simulink model "svm_Filter"  (R2023b)
settings: Solver=FixedStepAuto  StartTime=0.0  StopTime=0.08  FixedStep=0.5e-7  RelTol=1e-3
InitFcn:
  | TP=0.0002
  | Vdc=580
undefined symbols (not defined in the file): Ma
libraries: spsMosfetLib x6, spsSeriesRLCBranchLib x3, spsVoltageMeasurementLib x3, spsDCVoltageSourceLib x1, spsGroundLib x1, spsThreePhaseVIMeasurementLib x1, sps_lib x1, mcbcontrolslib x1, simulink_extras x1
settings Model: Creator=user  LastModifiedBy=user
settings DataIOCC: ReturnWorkspaceOutputs=off

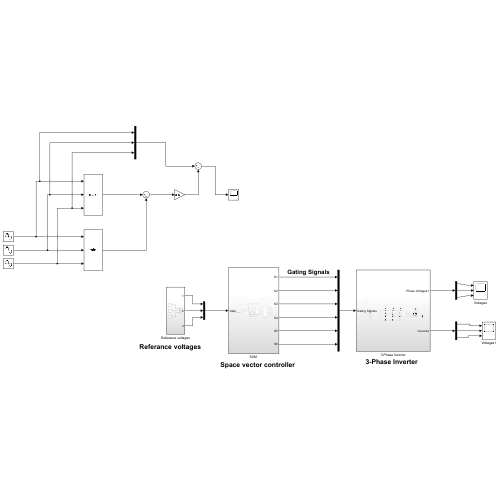
[thumbnail: Simulink's stored preview of the top-level diagram]
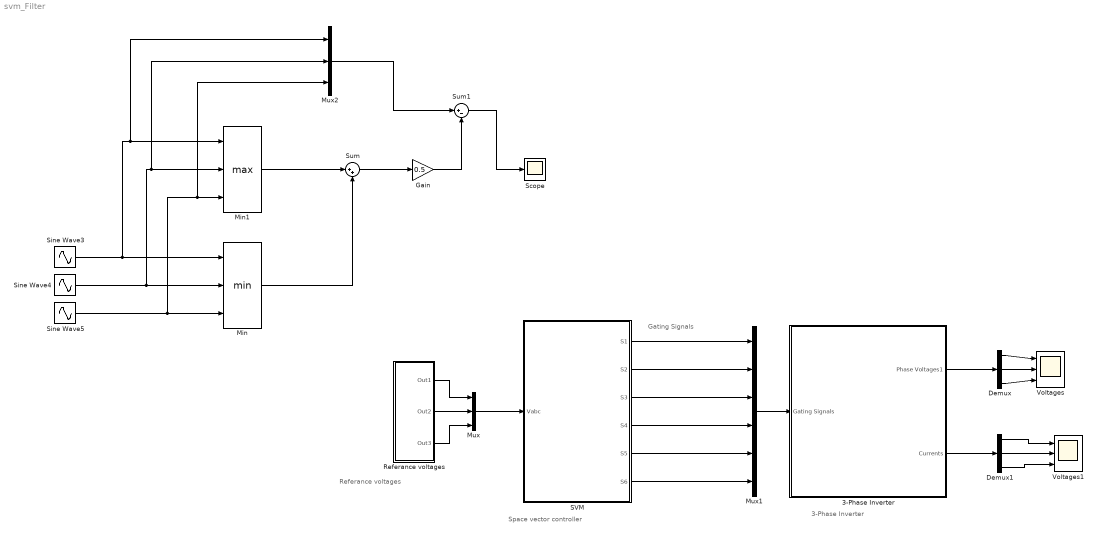
== system svm_Filter ==
  note: Gating Signals
  note: Space vector controller
  note: 3-Phase Inverter
  note: Referance voltages
  3-Phase Inverter : Subsystem
  Demux : Demux  Outputs=3
  Demux1 : Demux  Outputs=3
  Gain : Gain  Gain=0.5
  Min : MinMax  Inputs=3
  Min1 : MinMax  Function=max  Inputs=3
  Mux : Mux  Inputs=3
  Mux1 : Mux  Inputs=6
  Mux2 : Mux  Inputs=3
  Referance voltages : Subsystem
  "SVM " : Subsystem
  Scope : Scope
  Sine Wave3 : Sin  Amplitude=0.7*580  Frequency=100*pi  SampleTime=1e-6
  Sine Wave4 : Sin  Amplitude=0.7*580  Frequency=100*pi  Phase=120*pi/180  SampleTime=1e-6
  Sine Wave5 : Sin  Amplitude=0.7*580  Frequency=100*pi  Phase=240*pi/180  SampleTime=1e-6
  Sum : Sum  Inputs=|++
  Sum1 : Sum  Inputs=|+-
  Voltages : Scope  NumInputPorts=3
  Voltages1 : Scope  NumInputPorts=3
  wires:
  Mux/1 -> "SVM "/1(Vabc)
  "SVM "/1(S1) -> Mux1/1
  "SVM "/2(S2) -> Mux1/2
  "SVM "/3(S3) -> Mux1/3
  "SVM "/4(S4) -> Mux1/4
  "SVM "/5(S5) -> Mux1/5
  "SVM "/6(S6) -> Mux1/6
  Mux1/1 -> 3-Phase Inverter/1(Gating Signals)
  Demux/3 -> Voltages/3
  Demux/1 -> Voltages/1
  Demux/2 -> Voltages/2
  Demux1/2 -> Voltages1/2
  Demux1/3 -> Voltages1/3
  Demux1/1 -> Voltages1/1
  3-Phase Inverter/2(Currents) -> Demux1/1
  3-Phase Inverter/1(Phase Voltages1) -> Demux/1
  Sine Wave5/1 -> Mux2/3, Min1/3, Min/3
  Sine Wave3/1 -> Mux2/1, Min1/1, Min/1
  Sum/1 -> Gain/1
  Mux2/1 -> Sum1/1
  Sine Wave4/1 -> Mux2/2, Min1/2, Min/2
  Sum1/1 -> Scope/1
  Min1/1 -> Sum/1
  Gain/1 -> Sum1/2
  Min/1 -> Sum/2
  Referance voltages/1(Out1) -> Mux/1
  Referance voltages/2(Out2) -> Mux/2
  Referance voltages/3(Out3) -> Mux/3

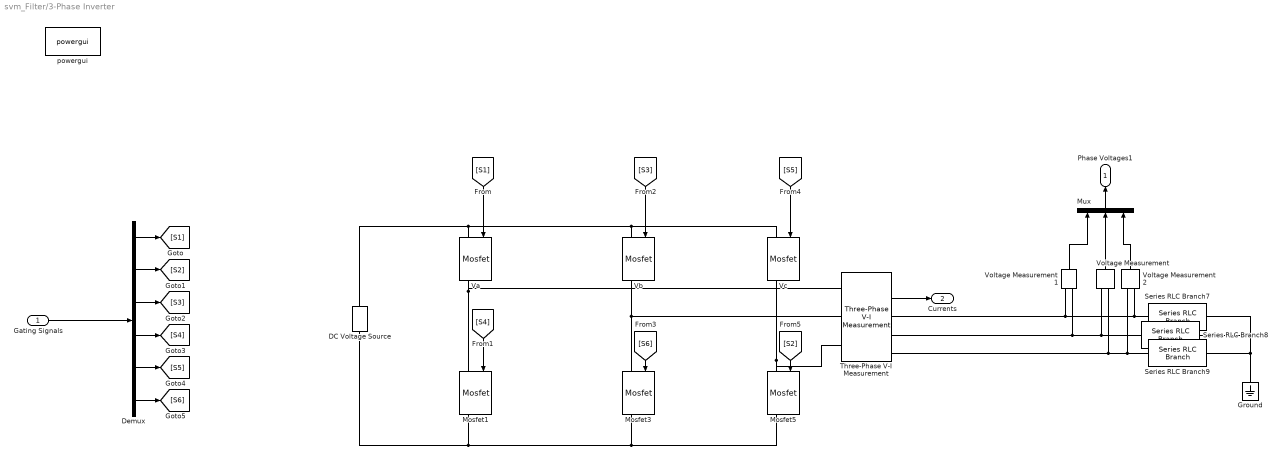
== system svm_Filter/3-Phase Inverter ==
  Gating Signals : Inport
  DC Voltage Source : spsDCVoltageSourceLib/DC Voltage Source  Amplitude=Vdc  Measurements=None
  Demux : Demux  Outputs=6
  Ground : spsGroundLib/Ground  LConnTagsString=a
  Mosfet1 : spsMosfetLib/Mosfet  Ron=0.1  Lon=0  Rd=0.01  Vfd=0  IC=0  Rs=1e5  Cs=inf  Measurements=on
  Mosfet3 : spsMosfetLib/Mosfet  Ron=0.1  Lon=0  Rd=0.01  Vfd=0  IC=0  Rs=1e5  Cs=inf  Measurements=on
  Mosfet5 : spsMosfetLib/Mosfet  Ron=0.1  Lon=0  Rd=0.01  Vfd=0  IC=0  Rs=1e5  Cs=inf  Measurements=on
  Mux : Mux  Inputs=3
  Series RLC Branch7 : spsSeriesRLCBranchLib/Series RLC Branch  LConnTagsString=__new0  RConnTagsString=__new0  BranchType=RL  Resistance=15  Inductance=10e-3  SetiL0=off  InitialCurrent=0  Capacitance=50e-6  Setx0=off  InitialVoltage=0  Measurements=None
  Series RLC Branch8 : spsSeriesRLCBranchLib/Series RLC Branch  LConnTagsString=__new0  RConnTagsString=__new0  BranchType=RL  Resistance=15  Inductance=10e-3  SetiL0=off  InitialCurrent=0  Capacitance=50e-6  Setx0=off  InitialVoltage=0  Measurements=None
  Series RLC Branch9 : spsSeriesRLCBranchLib/Series RLC Branch  LConnTagsString=__new0  RConnTagsString=__new0  BranchType=RL  Resistance=15  Inductance=10e-3  SetiL0=off  InitialCurrent=0  Capacitance=50e-6  Setx0=off  InitialVoltage=0  Measurements=None
  Three-Phase V-I Measurement : spsThreePhaseVIMeasurementLib/Three-Phase V-I Measurement  VoltageMeasurement=phase-to-phase  SetLabelV=off  LabelV=Vabc  Vpu=off  VpuLL=off  CurrentMeasurement=yes  SetLabelI=off  LabelI=Iabc  Ipu=off  Pbase=100e6  Vbase=500e3  OutputType=Complex  PhasorSimulation=off  PSBequivalent=0
  Va : spsMosfetLib/Mosfet  Ron=0.1  Lon=0  Rd=0.01  Vfd=0  IC=0  Rs=1e5  Cs=inf  Measurements=on
  Vb : spsMosfetLib/Mosfet  Ron=0.1  Lon=0  Rd=0.01  Vfd=0  IC=0  Rs=1e5  Cs=inf  Measurements=on
  Vc : spsMosfetLib/Mosfet  Ron=0.1  Lon=0  Rd=0.01  Vfd=0  IC=0  Rs=1e5  Cs=inf  Measurements=on
  Voltage Measurement : spsVoltageMeasurementLib/Voltage Measurement  PhasorSimulation=off  OutputType=Complex  PSBequivalent=0
  Voltage Measurement1 : spsVoltageMeasurementLib/Voltage Measurement  PhasorSimulation=off  OutputType=Complex  PSBequivalent=0
  Voltage Measurement2 : spsVoltageMeasurementLib/Voltage Measurement  PhasorSimulation=off  OutputType=Complex  PSBequivalent=0
  powergui : sps_lib/powergui  Priority=1  SimulationMode=Continuous  SampleTime=50e-6  frequency=60  Iterations=50  frequencyindice=0  Pbase=100e6  ErrMax=1e-4  UnitsV=kV  UnitsW=MW  buscounter=0  FunctionMessages=off  echomessages=off  EnableUseOfTLC=off  CurrentSourceSwitches=off  DisableSnubberDevices=off  DisableRonSwitches=off  DisableVfSwitches=off  DisplayEquations=off  AutomaticDiscreteSolvers=off  SolverType=Tustin/Backward Euler (TBE)  Interpol=off  ExternalGateDelay=off  methode=off  Ts=100  x0status=blocks  SPID=on  SwTol=0  HookPort=off  NonlinearTolerance=1e-4  nMaxIteration=100  ContinueOnMaxIteration=off  RestoreLinks=warning  ResistiveCurrentMeasurement=off  Frange=[0:2:500]  Ylog=off  Xlog=on  ShowGrid=off  save=off  variable=ZData  structure=0  ZoomFFT=off  StartTime=0.0  cycles=1  DisplayStyle=1  fundamental=60  FreqAxis=off  MaxFrequency=1000  frequencyindicesteady=1  RmsSteady=1  display=off
  Phase Voltages1 : Outport
  Currents : Outport  Port=2
  wires:
  [S6] -> Mosfet3/1
  [S2] -> Mosfet5/1
  [S3] -> Vb/1
  [S5] -> Vc/1
  [S1] -> Va/1
  [S4] -> Mosfet1/1
  Gating Signals/1 -> Demux/1
  Demux/1 -> [S1]
  Demux/2 -> [S2]
  Demux/3 -> [S3]
  Demux/4 -> [S4]
  Demux/5 -> [S5]
  Demux/6 -> [S6]
  Three-Phase V-I Measurement/2 -> Currents/1
  Voltage Measurement1/1 -> Mux/1
  Voltage Measurement/1 -> Mux/2
  Voltage Measurement2/1 -> Mux/3
  Mux/1 -> Phase Voltages1/1
  connections:
  Mosfet1/RConn1 -- DC Voltage Source/LConn1 -- Mosfet3/RConn1 -- Mosfet5/RConn1
  Va/LConn1 -- DC Voltage Source/RConn1 -- Vc/LConn1 -- Vb/LConn1
  Vc/RConn1 -- Three-Phase V-I Measurement/LConn3 -- Mosfet5/LConn1
  Vb/RConn1 -- Mosfet3/LConn1 -- Three-Phase V-I Measurement/LConn2
  Va/RConn1 -- Mosfet1/LConn1 -- Three-Phase V-I Measurement/LConn1
  Series RLC Branch7/LConn1 -- Voltage Measurement2/LConn2 -- Three-Phase V-I Measurement/RConn1 -- Voltage Measurement1/LConn1
  Series RLC Branch8/LConn1 -- Voltage Measurement1/LConn2 -- Three-Phase V-I Measurement/RConn2 -- Voltage Measurement/LConn1
  Series RLC Branch9/LConn1 -- Voltage Measurement/LConn2 -- Three-Phase V-I Measurement/RConn3 -- Voltage Measurement2/LConn1
  Ground/LConn1 -- Series RLC Branch9/RConn1 -- Series RLC Branch8/RConn1 -- Series RLC Branch7/RConn1

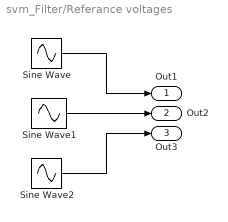
== system svm_Filter/Referance voltages ==
  Sine Wave : Sin  Amplitude=Ma  Frequency=100*pi  SampleTime=1e-6
  Sine Wave1 : Sin  Amplitude=Ma  Frequency=100*pi  Phase=-120*pi/180  SampleTime=1e-6
  Sine Wave2 : Sin  Amplitude=Ma  Frequency=100*pi  Phase=120*pi/180  SampleTime=1e-6
  Out1 : Outport
  Out2 : Outport  Port=2
  Out3 : Outport  Port=3
  wires:
  Sine Wave2/1 -> Out3/1
  Sine Wave/1 -> Out1/1
  Sine Wave1/1 -> Out2/1

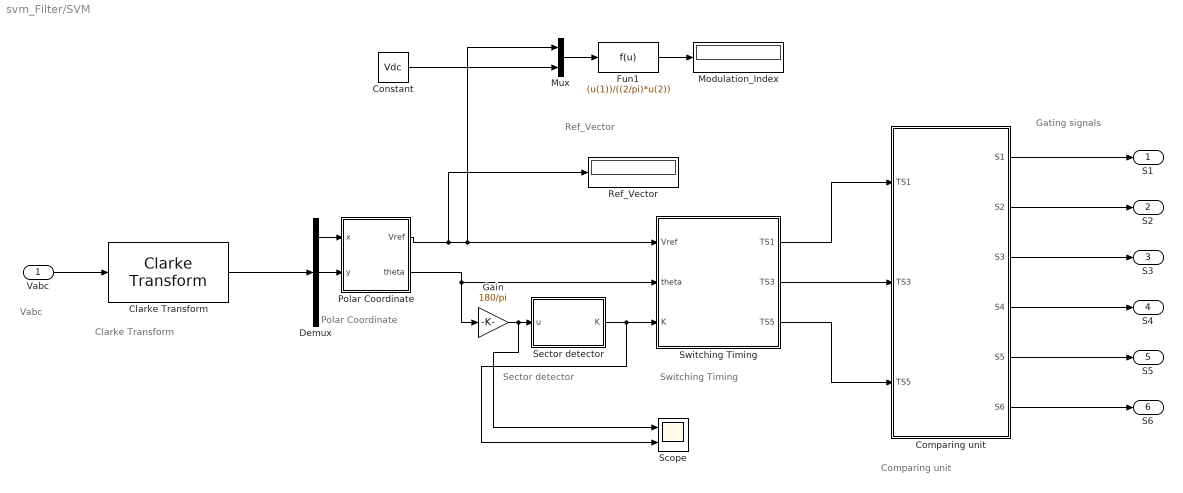
== system svm_Filter/SVM  ==
  note: Vabc
  note: Clarke Transform
  note: Polar Coordinate
  note: Sector detector
  note: Switching Timing
  note: Ref_Vector
  note: Gating signals
  note: Comparing unit
  Vabc : Inport
  Clarke Transform : mcbcontrolslib/Clarke Transform  VariantControl=Variant2  PhaseInput=Three inputs  EnPowerInv=off
      settings: LibrarySourceBlock=mcbhdllib/Controls/Math Transforms/Clarke Transform
  Comparing unit : Subsystem
  Constant : Constant  Value=Vdc
  Demux : Demux  Outputs=3
  Fun1 : Fcn  Expr=(u(1))/((2/pi)*u(2))
  Gain : Gain  Gain=180/pi
  Modulation_Index : Display
  Mux : Mux  Inputs=2
  Polar Coordinate : Subsystem
  Ref_Vector : Display
  Scope : Scope  NumInputPorts=2
  Sector detector : MATLAB Function  TreatAsAtomicUnit=on
  Switching Timing : Subsystem
  S1 : Outport
  S2 : Outport  Port=2
  S3 : Outport  Port=3
  S4 : Outport  Port=4
  S5 : Outport  Port=5
  S6 : Outport  Port=6
  wires:
  Vabc/1 -> Clarke Transform/1
  Demux/2 -> Polar Coordinate/2(y)
  Polar Coordinate/2(theta) -> Switching Timing/2(theta), Gain/1
  Gain/1 -> Scope/1, Sector detector/1(u)
  Sector detector/1(K) -> Scope/2, Switching Timing/3(K)
  Switching Timing/1(TS1) -> Comparing unit/1(TS1)
  Switching Timing/2(TS3) -> Comparing unit/2(TS3)
  Switching Timing/3(TS5) -> Comparing unit/3(TS5)
  Comparing unit/1(S1) -> S1/1
  Comparing unit/2(S2) -> S2/1
  Comparing unit/3(S3) -> S3/1
  Comparing unit/4(S4) -> S4/1
  Comparing unit/5(S5) -> S5/1
  Comparing unit/6(S6) -> S6/1
  Fun1/1 -> Modulation_Index/1
  Mux/1 -> Fun1/1
  Constant/1 -> Mux/2
  Polar Coordinate/1(Vref) -> Ref_Vector/1, Mux/1, Switching Timing/1(Vref)
  Clarke Transform/1 -> Demux/1
  Demux/1 -> Polar Coordinate/1(x)

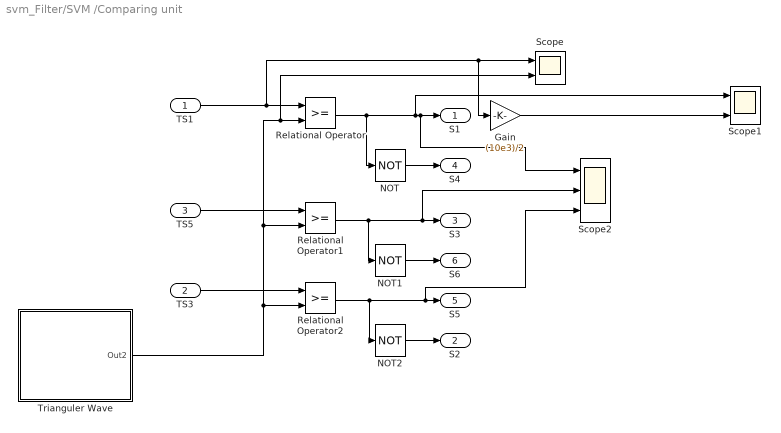
== system svm_Filter/SVM /Comparing unit ==
  TS1 : Inport
  TS3 : Inport  Port=2
  TS5 : Inport  Port=3
  Gain : Gain  Gain=(10e3)/2
  NOT : Logic  Operator=NOT  IconShape=distinctive  AllPortsSameDT=off  OutDataTypeStr=boolean
  NOT1 : Logic  Operator=NOT  IconShape=distinctive  AllPortsSameDT=off  OutDataTypeStr=boolean
  NOT2 : Logic  Operator=NOT  IconShape=distinctive  AllPortsSameDT=off  OutDataTypeStr=boolean
  Relational Operator : RelationalOperator  OutDataTypeStr=boolean  RndMeth=Simplest  InputSameDT=off
  Relational Operator1 : RelationalOperator  OutDataTypeStr=boolean  RndMeth=Simplest  InputSameDT=off
  Relational Operator2 : RelationalOperator  OutDataTypeStr=boolean  RndMeth=Simplest  InputSameDT=off
  Scope : Scope  NumInputPorts=2
  Scope1 : Scope  NumInputPorts=2
  Scope2 : Scope  NumInputPorts=3
  Trianguler Wave : Subsystem
  S1 : Outport
  S2 : Outport  Port=2
  S3 : Outport  Port=3
  S4 : Outport  Port=4
  S5 : Outport  Port=5
  S6 : Outport  Port=6
  wires:
  TS1/1 -> Gain/1, Scope/1, Relational Operator/1
  Relational Operator/1 -> NOT/1, Scope1/1, Scope2/1, S1/1
  NOT/1 -> S4/1
  TS5/1 -> Relational Operator1/1
  Relational Operator1/1 -> NOT1/1, Scope2/2, S3/1
  NOT1/1 -> S6/1
  TS3/1 -> Relational Operator2/1
  Relational Operator2/1 -> NOT2/1, Scope2/3, S5/1
  NOT2/1 -> S2/1
  Trianguler Wave/1(Out2) -> Relational Operator2/2, Relational Operator1/2, Scope/2, Relational Operator/2
  Gain/1 -> Scope1/2

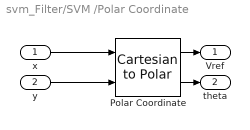
== system svm_Filter/SVM /Polar Coordinate ==
  x : Inport
  y : Inport  Port=2
  Polar Coordinate : simulink_extras/Transformations/Cartesian to Polar
  Vref : Outport
  theta : Outport  Port=2
  wires:
  y/1 -> Polar Coordinate/2
  Polar Coordinate/1 -> Vref/1
  Polar Coordinate/2 -> theta/1
  x/1 -> Polar Coordinate/1

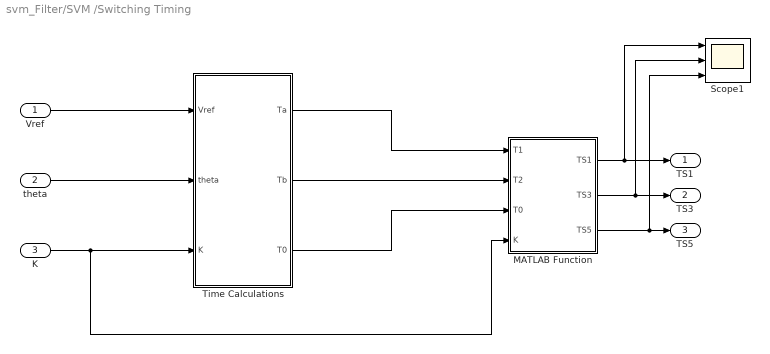
== system svm_Filter/SVM /Switching Timing ==
  Vref : Inport
  theta : Inport  Port=2
  K : Inport  Port=3
  MATLAB Function : MATLAB Function  TreatAsAtomicUnit=on
  Scope1 : Scope  NumInputPorts=3
  Time Calculations : Subsystem
  TS1 : Outport
  TS3 : Outport  Port=2
  TS5 : Outport  Port=3
  wires:
  Vref/1 -> Time Calculations/1(Vref)
  theta/1 -> Time Calculations/2(theta)
  K/1 -> MATLAB Function/4(K), Time Calculations/3(K)
  Time Calculations/1(Ta) -> MATLAB Function/1(T1)
  Time Calculations/2(Tb) -> MATLAB Function/2(T2)
  Time Calculations/3(T0) -> MATLAB Function/3(T0)
  MATLAB Function/1(TS1) -> Scope1/1, TS1/1
  MATLAB Function/2(TS3) -> Scope1/2, TS3/1
  MATLAB Function/3(TS5) -> Scope1/3, TS5/1

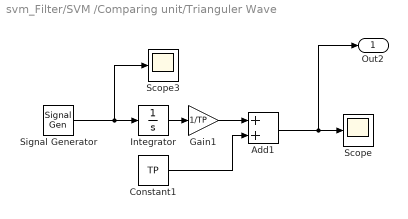
== system svm_Filter/SVM /Comparing unit/Trianguler Wave ==
  Add1 : Sum
  Constant1 : Constant  Value=TP
  Gain1 : Gain  Gain=1/TP
  Integrator : Integrator
  Scope : Scope
  Scope3 : Scope
  Signal Generator : SignalGenerator  WaveForm=square  Amplitude=TP  Frequency=1/(2*TP)
  Out2 : Outport  VectorParamsAs1DForOutWhenUnconnected=off
  wires:
  Constant1/1 -> Add1/2
  Integrator/1 -> Gain1/1
  Gain1/1 -> Add1/1
  Add1/1 -> Out2/1, Scope/1
  Signal Generator/1 -> Scope3/1, Integrator/1

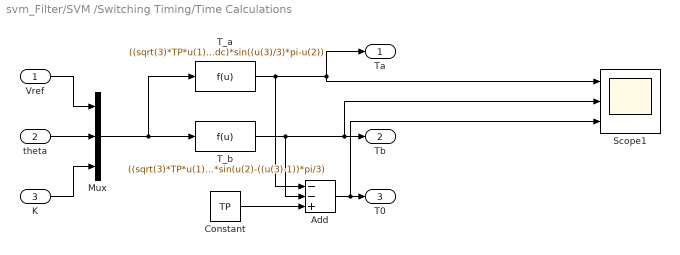
== system svm_Filter/SVM /Switching Timing/Time Calculations ==
  Vref : Inport
  theta : Inport  Port=2
  K : Inport  Port=3
  Add : Sum  Inputs=--+
  Constant : Constant  Value=TP
  Mux : Mux  Inputs=3
  Scope1 : Scope  NumInputPorts=3
  T_a : Fcn  Expr=((sqrt(3)*TP*u(1))/Vdc)*sin((u(3)/3)*pi-u(2))
  T_b : Fcn  Expr=((sqrt(3)*TP*u(1))/Vdc)*sin(u(2)-((u(3)-1))*pi/3)
  Ta : Outport
  Tb : Outport  Port=2
  T0 : Outport  Port=3
  wires:
  Mux/1 -> T_b/1, T_a/1
  Vref/1 -> Mux/1
  K/1 -> Mux/3
  theta/1 -> Mux/2
  T_a/1 -> Add/1, Scope1/1, Ta/1
  T_b/1 -> Add/2, Scope1/2, Tb/1
  Add/1 -> Scope1/3, T0/1
  Constant/1 -> Add/3

== matlab function svm_Filter/SVM /Switching Timing/MATLAB Function ==
  data: TS1 output; TS3 output; TS5 output; T1 input; T2 input; T0 input; K input
function [TS1,TS3,TS5]= fcn(T1,T2, T0, K)
switch K

    case 1
        TS1=T1+T2+T0/2;
        TS3=T2+T0/2;
        TS5=T0/2;
      
    case 2
        TS1=T1+T0/2;
        TS3=T1+T2+T0/2;
        TS5=T0/2;
     
    case 3
        TS1=T0/2;
        TS3=T1+T2+T0/2;
        TS5=T2+T0/2;
  
    case 4
        TS1=T0/2;
        TS3=T1+T0/2;
        TS5=T1+T2+T0/2;
        TS4=T1+T2+T0/2;
        TS6=T2+T0/2;
        TS2=T0/2;
    case 5
        TS1=T2+T0/2;
        TS3=T0/2;
        TS5=T1+T2+T0/2;
      
    case 6
        TS1=T1+T2+T0/2;
        TS3=T0/2;
        TS5=T1+T0/2;
      
    otherwise
        TS1=0;
        TS3=0;
        TS5=0;
      
end
end

== matlab function svm_Filter/SVM /Sector detector ==
  data: u input; K output
function K = fcn(u)
Sector=0;
if(u>=0&&u<60)
    Sector=1;
elseif(u>=60&&u<120)
    Sector=2;
elseif(u>=120&&u<180)
    Sector=3;
elseif(u>=-180&&u<-120)
    Sector=4;
elseif(u>=-120&&u<-60)
    Sector=5;
elseif(u>=-60&&u<0)
    Sector=6;
end
K = Sector;
